simulink model "trameMAC"  (R2012b)
settings: Solver=ode45  StartTime=0.0  StopTime=10.0  RelTol=1e-3
undefined symbols (not defined in the file): des
settings Model: Creator=Nora IZRI  LastModifiedBy=Nora IZRI

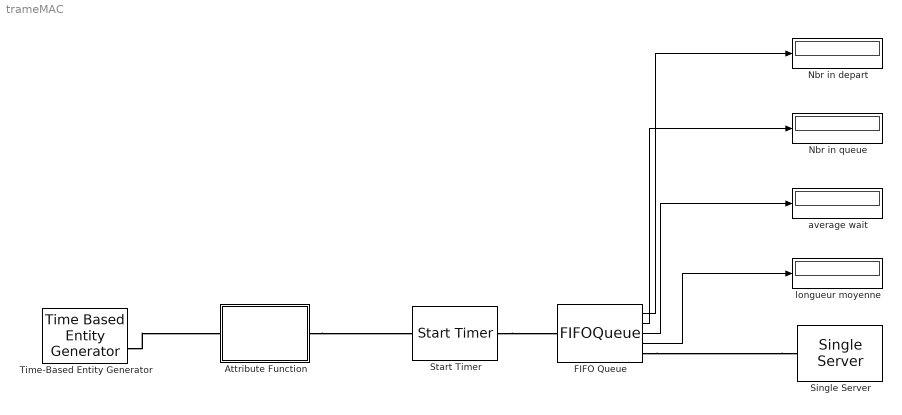
== system trameMAC ==
  Attribute Function : Subsystem  LoadFcn=des.afb.attributefunction_support(gcb,'LoadFcn');  StartFcn=des.afb.attributefunction_support(gcb,'StartFcn');  mask(Attribute Function){OutputNamePrefix=out_}
      mask prompts: OutputNamePrefix "Prefix name"
      settings: CopyFcn=des.afb.attributefunction_support(gcb,'CopyFcn');  OpenFcn=des.afb.attributefunction_support(gcb,'OpenFcn');  ErrorFcn=des.afb.error_redirect
      mask Help: slhelp(gcbh)
      mask Display: image(des_iconLoad('attribFunction.jpg'),'center');
  "FIFO Queue " : FIFOQueue  StatNumberDeparted=on  StatNumberInBlock=on  StatAverageWait=on  StatAverageQueueLength=on
      settings: OutputPortMap=o0,o1,o2,o3
  Nbr in depart : Display
  Nbr in queue : Display
  Single Server : SingleServer
  Start Timer : StartTimer
  Time-Based Entity Generator : TimeBasedEntityGenerator  Distribution=Exponential  StatNumberDeparted=on
  average wait : Display
  longueur moyenne : Display
  wires:
  "FIFO Queue "/4 -> longueur moyenne/1
  "FIFO Queue "/3 -> average wait/1
  "FIFO Queue "/2 -> Nbr in queue/1
  "FIFO Queue "/1 -> Nbr in depart/1
  connections:
  Time-Based Entity Generator/RConn1 -- Attribute Function/LConn1
  Attribute Function/RConn1 -- Start Timer/LConn1
  Start Timer/RConn1 -- "FIFO Queue "/LConn1
  "FIFO Queue "/RConn1 -- Single Server/LConn1

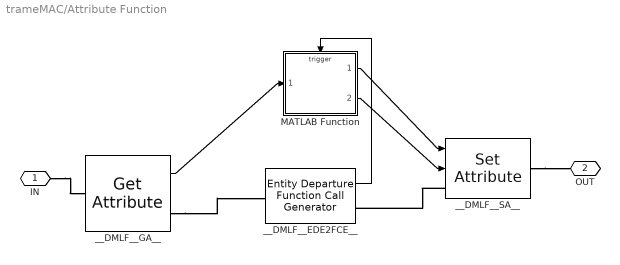
== system trameMAC/Attribute Function ==
  MATLAB Function : MATLAB Function  TreatAsAtomicUnit=on
  __DMLF__EDE2FCE__ : EntityDepartureFunctionCallGenerator  TimingFunctionCallF1=Before entity departure  IsInsideAFB=on
  __DMLF__GA__ : GetAttribute  AttributeSendTiming=Before entity departure  EvaluatedDefaultAttributeValue={ []}  IsInsideAFB=on
      settings: OutputPortMap=o1
  __DMLF__SA__ : SetAttribute  AttributeName=Attribute1|Attribute2  AttributeFrom=Signal port|Signal port  AttributeValue=1|1  AttributeTreatAsVector=1|1  EvaluatedAttributeValue={ []; [] }  IsInsideAFB=on
      settings: InputPortMap=u0,u1
  IN : PMIOPort  Port=1  Side=Left
  OUT : PMIOPort  Port=2  Side=Right
  wires:
  __DMLF__EDE2FCE__/1 -> MATLAB Function/Trigger
  __DMLF__GA__/1 -> MATLAB Function/1(Attribute1)
  MATLAB Function/1(out_Attribute1) -> __DMLF__SA__/1
  MATLAB Function/2(out_Attribute2) -> __DMLF__SA__/2
  connections:
  __DMLF__SA__/LConn1 -- __DMLF__EDE2FCE__/RConn1
  __DMLF__GA__/RConn1 -- __DMLF__EDE2FCE__/LConn1
  IN/RConn1 -- __DMLF__GA__/LConn1
  __DMLF__SA__/RConn1 -- OUT/RConn1

== matlab function trameMAC/Attribute Function/MATLAB Function ==
  data: Attribute1 input; out_Attribute1 output; out_Attribute2 output
  events: trigger input FUNCTION_CALL_EVENT
function [out_Attribute1, out_Attribute2] = fcn(Attribute1)
%FCN    Access and modify attributes with MATLAB 
% 
% Input arguments must match the attribute names.
% Output arguments must be out_<AttributeName>,
% e.g., out_ServiceTime where ServiceTime is the attribute name.
% 
% The output attribute will be created if it is not present.
%

out_Attribute1 = Attribute1 + 1;
out_Attribute2 = Attribute1*2;
